simulink library "findUnitVectors_ul"  (R2018b)
settings: Solver=VariableStepAuto  StartTime=0.0  StopTime=10.0  RelTol=1e-3
settings Model: Creator=mcobb  LastModifiedBy=MAE-NCSUCORE
settings DebuggingCC: LibraryContextMissingDiagnostic=none
settings SFSimCC: SimUseLocalCustomCode=off
settings RTWCC: RTWUseLocalCustomCode=off

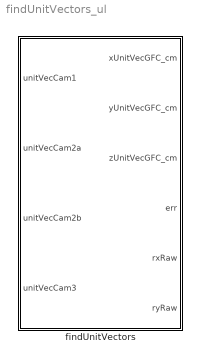
== system findUnitVectors_ul ==
  findUnitVectors : Subsystem  mask{sideSeparation_cm=0, bottomASeparation_cm=0, bottomBSeparation_cm=0, DSB=[0 0 0], DBL=[0 0 0]}
      mask prompts: sideSeparation_cm "Side Dot Set Separation Distance [cm]"; bottomASeparation_cm "Bottom Dot Set A Separation Distance [cm]"; bottomBSeparation_cm "Bottom Dot Set B Separation Distance [cm]"; DSB "x Unit Vec Left Pseudo Inverse"; DBL "y Unit Vec Left Pseudo Inverse"

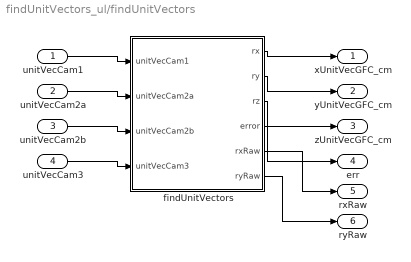
== system findUnitVectors_ul/findUnitVectors ==
  unitVecCam1 : Inport
  unitVecCam2a : Inport  Port=2
  unitVecCam2b : Inport  Port=3
  unitVecCam3 : Inport  Port=4
  findUnitVectors : MATLAB Function  TreatAsAtomicUnit=on
  xUnitVecGFC_cm : Outport  PortDimensions=[3 1]
  yUnitVecGFC_cm : Outport  Port=2  PortDimensions=[3 1]
  zUnitVecGFC_cm : Outport  Port=3  PortDimensions=[3 1]
  err : Outport  Port=4  PortDimensions=1
  rxRaw : Outport  Port=5
  ryRaw : Outport  Port=6
  wires:
  unitVecCam1/1 -> findUnitVectors/1(unitVecCam1)
  findUnitVectors/1(rx) -> xUnitVecGFC_cm/1
  findUnitVectors/2(ry) -> yUnitVecGFC_cm/1
  findUnitVectors/3(rz) -> zUnitVecGFC_cm/1
  findUnitVectors/4(error) -> err/1
  unitVecCam2a/1 -> findUnitVectors/2(unitVecCam2a)
  unitVecCam2b/1 -> findUnitVectors/3(unitVecCam2b)
  unitVecCam3/1 -> findUnitVectors/4(unitVecCam3)
  findUnitVectors/5(rxRaw) -> rxRaw/1
  findUnitVectors/6(ryRaw) -> ryRaw/1

== matlab function findUnitVectors_ul/findUnitVectors/findUnitVectors ==
  data: unitVecCam1 input size=[1 2]; unitVecCam2a input size=[1 2]; rx output size=[3,1]; ry output size=[3,1]; unitVecCam2b input size=[1 2]; unitVecCam3 input size=[1 2]; rz output size=[3,1]; DSB parameter size=[3,4]; DBL parameter size=[3,4]; bottomASeparation_cm parameter size=1; error output size=1; bottomBSeparation_cm parameter size=1; sideSeparation_cm parameter size=1; rxRaw output; ryRaw output
function [rx,ry,rz,error,rxRaw,ryRaw] = fcn(unitVecCam1,unitVecCam2a,unitVecCam2b,...
    unitVecCam3,DSB,DBL, bottomASeparation_cm, bottomBSeparation_cm, sideSeparation_cm)
%#codegen
[rx,ry,rz,error,rxRaw,ryRaw] = findUnitVectors(unitVecCam1,unitVecCam2a,...
    unitVecCam2b,unitVecCam3,sideSeparation_cm,bottomASeparation_cm,bottomBSeparation_cm,DSB,DBL);
end
